simulink model "Model"  (R2020b)
settings: Solver=VariableStepAuto  StartTime=0.0  StopTime=20  MaxStep=0.1  RelTol=1e-1
values from neighbouring files (symbols this model uses):
  D = [0 ... (first row only)    [Data_clean.m]
  g = 9.81    [Data_clean.m]
  k_cart = 0.0113    [Data_clean.m]
  L = 5    [Data_clean.m]
  m = 12000    [Data_clean.m]
  M = 1000    [Data_clean.m]
  Ts = 0.1    [Data_clean.m]
undefined symbols (not defined in the file or in its folder): blk, Discrete, iA, isLTV, lastPcov, lastu, lastx, MDscale, mpc1_plant, MVscale, nCC, nu, nud, nv, nxp, ny, nym, p, RMVscale, Time, ts, uoff, X, xoff, Y, Yscale, Z
libraries: sm_lib x76, mpcsigdimcheck_private x76, nesl_utility x12, ctrlSharedLib x8, simulink_extras x5, mpclib x1
(part 1 of 8)
settings Model: Creator=kashirin.as  LastModifiedBy=LASK
settings SolverCC: AlgebraicLoopSolver=LineSearch
settings DebuggingCC: UnderSpecifiedDimensionMsg=warning
settings ConfigComp: PLC_TargetIDE=tiaportal_double

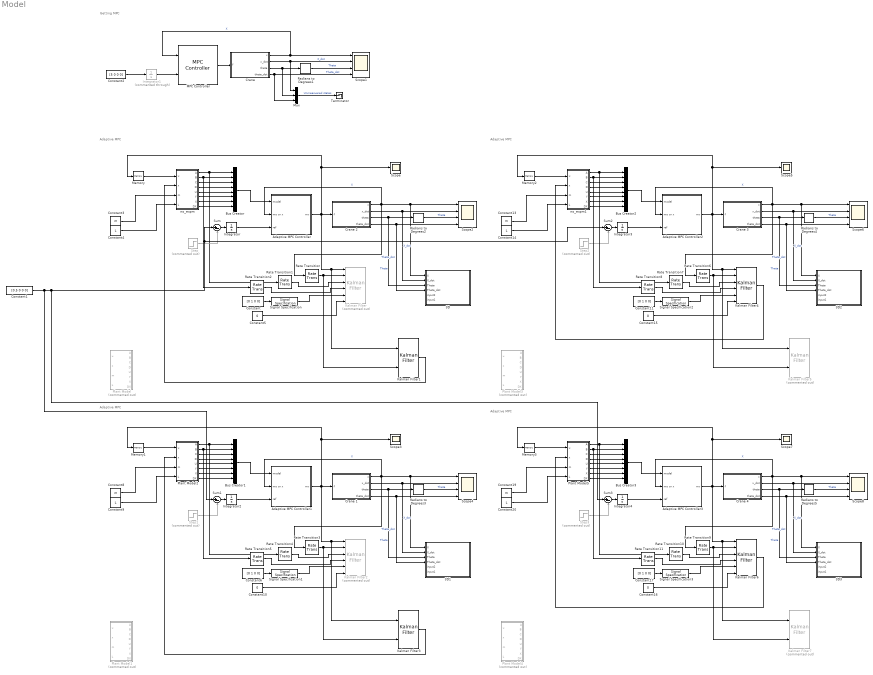
== system Model ==
  note: Getting MPC
  note: Adaptive MPC
  note: Adaptive MPC
  note: Adaptive MPC
  note: Adaptive MPC
  3D : Subsystem
  3D1 : Subsystem
  3D2 : Subsystem
  3D3 : Subsystem
  Adaptive MPC Controller : Subsystem  AncestorBlock=mpclib/Adaptive MPC Controller  SCDEnableBlockLinearizationSpecification=on  InitFcn=ampcblock_InitFcn  StartFcn=ampcblock_StartFcn  mask(Adaptive MPC){mpcobj=mpc1, x0=, enable_value=0, updateMPCinCallerWorkspace=on, md_inport=off, mv_inport=off, uref_inport=off, return_cost=off, return_mvseq=off, return_qpstatus=off, return_xseq=off, return_state=off, return_ovseq=off, state_inport=off, isltv_plant=off, umin_inport=off, umax_inport=off, ymin_inport=off, ymax_inport=off, cc_inport=off, ywt_inport=off, uwt_inport=off, duwt_inport=off, rhoeps_inport=off, pm_inport=off, MaximumP=10, HorizonChoice=FixedHorizon, BlockDataType=double, SampleTimeInherited=off, switch_inport=off}
      mask prompts: mpcobj "MPC:general:BlgAMPC"; x0 "MPC:general:BlgState"; enable_value "Value enabling optimization"; updateMPCinCallerWorkspace "Update MPC object in caller workspace"; md_inport "MPC:general:BlgMD"; mv_inport "MPC:general:BlgEXTMV"; uref_inport "MPC:general:BlgMVTARGET"; return_cost "MPC:general:BlgCOST"; return_mvseq "MPC:general:BlgMVSEQ"; return_qpstatus "MPC:general:BlgQPSTATUS"; return_xseq "MPC:general:BlgXSEQ"; return_state "MPC:general:BlgESTSTATE"; return_ovseq "MPC:general:BlgOVSEQ"; state_inport "MPC:general:BlgXKK"; isltv_plant "MPC:general:BlgLTV"; umin_inport "MPC:general:BlgMVMin"; umax_inport "MPC:general:BlgMVMax"; ymin_inport "MPC:general:BlgOVMin"; ymax_inport "MPC:general:BlgOVMax"; cc_inport "Custom constraints (E, F, G, S)"; ywt_inport "MPC:general:BlgYWT"; uwt_inport "MPC:general:BlgUWT"; duwt_inport "MPC:general:BlgDUWT"; rhoeps_inport "MPC:general:BlgECRWT"; pm_inport "MPC:general:BlgPM"; MaximumP "MPC:general:BlgMaximumP"; HorizonChoice "Simulink:Variants:LabelComboBox"; BlockDataType "MPC:general:BlgDATATYPE"; SampleTimeInherited "MPC:general:BlgTS"; switch_inport "MPC:general:BlgSWITCH"
      mask help: MPC:utility:MaskDescAdaptiveMPC1
      mask init:
      | [blk,ts,A,B,C,D,isQP,strmoorx,nmoorx,nu,nv,ny,nx,nym,nud,...
      |     degrees,lastPcov,H,Hinv,Linv,iA,Ac,Kx,Ku1,Kut,Kr,Kv,...
      |     Mlim,Mx,Mu1,Mv,z_degrees,utarget,...
      |     lastx,lastu,p,xoff,uoff,yoff,voff,myoff,no_md,no_ref,...
      |     CustomSolver,CustomSolverCodeGen,UseSuboptimalSolution,...
      |     UseActiveSetSolver,ASOptions,IPOptions,...
      |     nxQP,openloopflag,no_ym,no_mv,no_uref,...
      |     no_umin,no_umax,no_ymin,no_ymax,no_cc,...
      |     no_switch,CustomEstimation,...
      |     no_ywt, no_uwt, no_duwt, no_rhoeps,...
      |     Wy,Wdu,Jm,SuJm,Su1,Sx,Hv,Wu,I1,...
      |     isAdaptive, isLTV, Mrows, nCC, Ecc, Fcc, Scc, Gcc, Cid, Did, ...
      |     nxp, nup, nxid, mvindex, mdindex, unindex, myindex, ...
      |     Uscale, Yscale, MVscale, MDscale, ...
      |     RYscale,RMYscale,RMVscale,RMDscale,no_p,no_m,p0,m] = ampcblock_MaskInitFcnParameter();
      | ampcblock_MaskInitFcnResize(gcb,nv,nu,ny,nCC);
      mask Help: eval('mpcCSHelp(''MPCmaskAdaptive'',''HelpBrowser'')');
      mask Callback pm_inport: mpcblocks_callbackPM(gcb);
      mask TypeOptions HorizonChoice: MPC/optimizer/LabelModeActiveChoice
      mask DialogControl mpcobj Prompt: Adaptive MPC Controller
      mask DialogControl x0 Prompt: Initial Controller State
      mask DialogControl Container5 Prompt: MPC:general:BlgTab1
      mask DialogControl Container6 Prompt: MPC:general:BlgBox11
      mask DialogControl md_inport Prompt: Measured disturbance (md)
      mask DialogControl mv_inport Prompt: External manipulated variable (ext.mv)
      mask DialogControl uref_inport Prompt: Targets for manipulated variables (mv.target)
      mask DialogControl Container7 Prompt: MPC:general:BlgBox12
      mask DialogControl return_cost Prompt: Optimal cost (cost)
      mask DialogControl return_mvseq Prompt: Optimal control sequence (mv.seq)
      mask DialogControl return_qpstatus Prompt: Optimization status (qp.status)
      mask DialogControl return_xseq Prompt: Optimal state sequence (x.seq)
      mask DialogControl return_state Prompt: Estimated controller states (est.state)
      mask DialogControl return_ovseq Prompt: Optimal output sequence (y.seq)
      mask DialogControl Container16 Prompt: MPC:general:BlgBox13
      mask DialogControl state_inport Prompt: Use custom state estimation instead of using the built-in Kalman filter (x[k|k])
      mask DialogControl Container9 Prompt: MPC:general:BlgTab2
      mask DialogControl Container19 Prompt: MPC:general:BlgBox20
      mask DialogControl isltv_plant Prompt: Linear Time-Varying (LTV) plants (model expects 3-D signals)
      mask DialogControl Container10 Prompt: MPC:general:BlgBox21
      mask DialogControl umin_inport Prompt: Lower MV limits (umin)
      mask DialogControl umax_inport Prompt: Upper MV limits (umax)
      mask DialogControl ymin_inport Prompt: Lower OV limits (ymin)
      mask DialogControl ymax_inport Prompt: Upper OV limits (ymax)
      mask DialogControl Container11 Prompt: MPC:general:BlgBox22
      mask DialogControl ywt_inport Prompt: OV weights (y.wt)
      mask DialogControl uwt_inport Prompt: MV weights (u.wt)
      mask DialogControl duwt_inport Prompt: MVRate weights (du.wt)
      mask DialogControl rhoeps_inport Prompt: Slack variable weight (ecr.wt)
      mask DialogControl Container17 Prompt: Prediction and Control Horizons
      mask DialogControl pm_inport Prompt: Adjust prediction horizon (p) and control horizon (m) at run time
      mask DialogControl MaximumP Prompt: Maximum prediction horizon
      mask DialogControl HorizonChoice Prompt: Label mode active choice:
      mask DialogControl Container13 Prompt: MPC:general:BlgTab3
      mask DialogControl Container14 Prompt: MPC:general:BlgBox31
      mask DialogControl BlockDataType Prompt: Block Data Type
      mask DialogControl Container15 Prompt: MPC:general:BlgBox32
      mask DialogControl SampleTimeInherited Prompt: Inherit sample time (must be the same as controller sample time)
      mask DialogControl Container18 Prompt: MPC:general:BlgBox33
      mask DialogControl switch_inport Prompt: Use external signal to enable or disable optimization (switch)
      mask Display:
      | fprintf('Adaptive\nMPC');
      | port_label('output', 1, 'mv')
      | port_label('input', 1, 'model')
      | port_label('input', 2, 'mo')
      | port_label('input', 3, 'ref')
  Adaptive MPC Controller1 : Subsystem  AncestorBlock=mpclib/Adaptive MPC Controller  SCDEnableBlockLinearizationSpecification=on  InitFcn=ampcblock_InitFcn  StartFcn=ampcblock_StartFcn  mask(Adaptive MPC){mpcobj=mpc1, x0=, enable_value=0, updateMPCinCallerWorkspace=on, md_inport=off, mv_inport=off, uref_inport=off, return_cost=off, return_mvseq=off, return_qpstatus=off, return_xseq=off, return_state=off, return_ovseq=off, state_inport=off, isltv_plant=off, umin_inport=off, umax_inport=off, ymin_inport=off, ymax_inport=off, cc_inport=off, ywt_inport=off, uwt_inport=off, duwt_inport=off, rhoeps_inport=off, pm_inport=off, MaximumP=10, HorizonChoice=FixedHorizon, BlockDataType=double, SampleTimeInherited=off, switch_inport=off}
      mask prompts: mpcobj "MPC:general:BlgAMPC"; x0 "MPC:general:BlgState"; enable_value "Value enabling optimization"; updateMPCinCallerWorkspace "Update MPC object in caller workspace"; md_inport "MPC:general:BlgMD"; mv_inport "MPC:general:BlgEXTMV"; uref_inport "MPC:general:BlgMVTARGET"; return_cost "MPC:general:BlgCOST"; return_mvseq "MPC:general:BlgMVSEQ"; return_qpstatus "MPC:general:BlgQPSTATUS"; return_xseq "MPC:general:BlgXSEQ"; return_state "MPC:general:BlgESTSTATE"; return_ovseq "MPC:general:BlgOVSEQ"; state_inport "MPC:general:BlgXKK"; isltv_plant "MPC:general:BlgLTV"; umin_inport "MPC:general:BlgMVMin"; umax_inport "MPC:general:BlgMVMax"; ymin_inport "MPC:general:BlgOVMin"; ymax_inport "MPC:general:BlgOVMax"; cc_inport "Custom constraints (E, F, G, S)"; ywt_inport "MPC:general:BlgYWT"; uwt_inport "MPC:general:BlgUWT"; duwt_inport "MPC:general:BlgDUWT"; rhoeps_inport "MPC:general:BlgECRWT"; pm_inport "MPC:general:BlgPM"; MaximumP "MPC:general:BlgMaximumP"; HorizonChoice "Simulink:Variants:LabelComboBox"; BlockDataType "MPC:general:BlgDATATYPE"; SampleTimeInherited "MPC:general:BlgTS"; switch_inport "MPC:general:BlgSWITCH"
      mask help: MPC:utility:MaskDescAdaptiveMPC1
      mask init: same as Model/Adaptive MPC Controller
      mask Help: eval('mpcCSHelp(''MPCmaskAdaptive'',''HelpBrowser'')');
      mask Callback pm_inport: mpcblocks_callbackPM(gcb);
      mask TypeOptions HorizonChoice: MPC/optimizer/LabelModeActiveChoice
      mask DialogControl mpcobj Prompt: Adaptive MPC Controller
      mask DialogControl x0 Prompt: Initial Controller State
      mask DialogControl Container5 Prompt: MPC:general:BlgTab1
      mask DialogControl Container6 Prompt: MPC:general:BlgBox11
      mask DialogControl md_inport Prompt: Measured disturbance (md)
      mask DialogControl mv_inport Prompt: External manipulated variable (ext.mv)
      mask DialogControl uref_inport Prompt: Targets for manipulated variables (mv.target)
      mask DialogControl Container7 Prompt: MPC:general:BlgBox12
      mask DialogControl return_cost Prompt: Optimal cost (cost)
      mask DialogControl return_mvseq Prompt: Optimal control sequence (mv.seq)
      mask DialogControl return_qpstatus Prompt: Optimization status (qp.status)
      mask DialogControl return_xseq Prompt: Optimal state sequence (x.seq)
      mask DialogControl return_state Prompt: Estimated controller states (est.state)
      mask DialogControl return_ovseq Prompt: Optimal output sequence (y.seq)
      mask DialogControl Container16 Prompt: MPC:general:BlgBox13
      mask DialogControl state_inport Prompt: Use custom state estimation instead of using the built-in Kalman filter (x[k|k])
      mask DialogControl Container9 Prompt: MPC:general:BlgTab2
      mask DialogControl Container19 Prompt: MPC:general:BlgBox20
      mask DialogControl isltv_plant Prompt: Linear Time-Varying (LTV) plants (model expects 3-D signals)
      mask DialogControl Container10 Prompt: MPC:general:BlgBox21
      mask DialogControl umin_inport Prompt: Lower MV limits (umin)
      mask DialogControl umax_inport Prompt: Upper MV limits (umax)
      mask DialogControl ymin_inport Prompt: Lower OV limits (ymin)
      mask DialogControl ymax_inport Prompt: Upper OV limits (ymax)
      mask DialogControl Container11 Prompt: MPC:general:BlgBox22
      mask DialogControl ywt_inport Prompt: OV weights (y.wt)
      mask DialogControl uwt_inport Prompt: MV weights (u.wt)
      mask DialogControl duwt_inport Prompt: MVRate weights (du.wt)
      mask DialogControl rhoeps_inport Prompt: Slack variable weight (ecr.wt)
      mask DialogControl Container17 Prompt: Prediction and Control Horizons
      mask DialogControl pm_inport Prompt: Adjust prediction horizon (p) and control horizon (m) at run time
      mask DialogControl MaximumP Prompt: Maximum prediction horizon
      mask DialogControl HorizonChoice Prompt: Label mode active choice:
      mask DialogControl Container13 Prompt: MPC:general:BlgTab3
      mask DialogControl Container14 Prompt: MPC:general:BlgBox31
      mask DialogControl BlockDataType Prompt: Block Data Type
      mask DialogControl Container15 Prompt: MPC:general:BlgBox32
      mask DialogControl SampleTimeInherited Prompt: Inherit sample time (must be the same as controller sample time)
      mask DialogControl Container18 Prompt: MPC:general:BlgBox33
      mask DialogControl switch_inport Prompt: Use external signal to enable or disable optimization (switch)
      mask Display:
      | fprintf('Adaptive\nMPC');
      | port_label('output', 1, 'mv')
      | port_label('input', 1, 'model')
      | port_label('input', 2, 'mo')
      | port_label('input', 3, 'ref')
  Adaptive MPC Controller2 : Subsystem  AncestorBlock=mpclib/Adaptive MPC Controller  SCDEnableBlockLinearizationSpecification=on  InitFcn=ampcblock_InitFcn  StartFcn=ampcblock_StartFcn  mask(Adaptive MPC){mpcobj=mpc1, x0=, enable_value=0, updateMPCinCallerWorkspace=on, md_inport=off, mv_inport=off, uref_inport=off, return_cost=off, return_mvseq=off, return_qpstatus=off, return_xseq=off, return_state=off, return_ovseq=off, state_inport=off, isltv_plant=off, umin_inport=off, umax_inport=off, ymin_inport=off, ymax_inport=off, cc_inport=off, ywt_inport=off, uwt_inport=off, duwt_inport=off, rhoeps_inport=off, pm_inport=off, MaximumP=10, HorizonChoice=FixedHorizon, BlockDataType=double, SampleTimeInherited=off, switch_inport=off}
      mask prompts: mpcobj "MPC:general:BlgAMPC"; x0 "MPC:general:BlgState"; enable_value "Value enabling optimization"; updateMPCinCallerWorkspace "Update MPC object in caller workspace"; md_inport "MPC:general:BlgMD"; mv_inport "MPC:general:BlgEXTMV"; uref_inport "MPC:general:BlgMVTARGET"; return_cost "MPC:general:BlgCOST"; return_mvseq "MPC:general:BlgMVSEQ"; return_qpstatus "MPC:general:BlgQPSTATUS"; return_xseq "MPC:general:BlgXSEQ"; return_state "MPC:general:BlgESTSTATE"; return_ovseq "MPC:general:BlgOVSEQ"; state_inport "MPC:general:BlgXKK"; isltv_plant "MPC:general:BlgLTV"; umin_inport "MPC:general:BlgMVMin"; umax_inport "MPC:general:BlgMVMax"; ymin_inport "MPC:general:BlgOVMin"; ymax_inport "MPC:general:BlgOVMax"; cc_inport "Custom constraints (E, F, G, S)"; ywt_inport "MPC:general:BlgYWT"; uwt_inport "MPC:general:BlgUWT"; duwt_inport "MPC:general:BlgDUWT"; rhoeps_inport "MPC:general:BlgECRWT"; pm_inport "MPC:general:BlgPM"; MaximumP "MPC:general:BlgMaximumP"; HorizonChoice "Simulink:Variants:LabelComboBox"; BlockDataType "MPC:general:BlgDATATYPE"; SampleTimeInherited "MPC:general:BlgTS"; switch_inport "MPC:general:BlgSWITCH"
      mask help: MPC:utility:MaskDescAdaptiveMPC1
      mask init: same as Model/Adaptive MPC Controller
      mask Help: eval('mpcCSHelp(''MPCmaskAdaptive'',''HelpBrowser'')');
      mask Callback pm_inport: mpcblocks_callbackPM(gcb);
      mask TypeOptions HorizonChoice: MPC/optimizer/LabelModeActiveChoice
      mask DialogControl mpcobj Prompt: Adaptive MPC Controller
      mask DialogControl x0 Prompt: Initial Controller State
      mask DialogControl Container5 Prompt: MPC:general:BlgTab1
      mask DialogControl Container6 Prompt: MPC:general:BlgBox11
      mask DialogControl md_inport Prompt: Measured disturbance (md)
      mask DialogControl mv_inport Prompt: External manipulated variable (ext.mv)
      mask DialogControl uref_inport Prompt: Targets for manipulated variables (mv.target)
      mask DialogControl Container7 Prompt: MPC:general:BlgBox12
      mask DialogControl return_cost Prompt: Optimal cost (cost)
      mask DialogControl return_mvseq Prompt: Optimal control sequence (mv.seq)
      mask DialogControl return_qpstatus Prompt: Optimization status (qp.status)
      mask DialogControl return_xseq Prompt: Optimal state sequence (x.seq)
      mask DialogControl return_state Prompt: Estimated controller states (est.state)
      mask DialogControl return_ovseq Prompt: Optimal output sequence (y.seq)
      mask DialogControl Container16 Prompt: MPC:general:BlgBox13
      mask DialogControl state_inport Prompt: Use custom state estimation instead of using the built-in Kalman filter (x[k|k])
      mask DialogControl Container9 Prompt: MPC:general:BlgTab2
      mask DialogControl Container19 Prompt: MPC:general:BlgBox20
      mask DialogControl isltv_plant Prompt: Linear Time-Varying (LTV) plants (model expects 3-D signals)
      mask DialogControl Container10 Prompt: MPC:general:BlgBox21
      mask DialogControl umin_inport Prompt: Lower MV limits (umin)
      mask DialogControl umax_inport Prompt: Upper MV limits (umax)
      mask DialogControl ymin_inport Prompt: Lower OV limits (ymin)
      mask DialogControl ymax_inport Prompt: Upper OV limits (ymax)
      mask DialogControl Container11 Prompt: MPC:general:BlgBox22
      mask DialogControl ywt_inport Prompt: OV weights (y.wt)
      mask DialogControl uwt_inport Prompt: MV weights (u.wt)
      mask DialogControl duwt_inport Prompt: MVRate weights (du.wt)
      mask DialogControl rhoeps_inport Prompt: Slack variable weight (ecr.wt)
      mask DialogControl Container17 Prompt: Prediction and Control Horizons
      mask DialogControl pm_inport Prompt: Adjust prediction horizon (p) and control horizon (m) at run time
      mask DialogControl MaximumP Prompt: Maximum prediction horizon
      mask DialogControl HorizonChoice Prompt: Label mode active choice:
      mask DialogControl Container13 Prompt: MPC:general:BlgTab3
      mask DialogControl Container14 Prompt: MPC:general:BlgBox31
      mask DialogControl BlockDataType Prompt: Block Data Type
      mask DialogControl Container15 Prompt: MPC:general:BlgBox32
      mask DialogControl SampleTimeInherited Prompt: Inherit sample time (must be the same as controller sample time)
      mask DialogControl Container18 Prompt: MPC:general:BlgBox33
      mask DialogControl switch_inport Prompt: Use external signal to enable or disable optimization (switch)
      mask Display:
      | fprintf('Adaptive\nMPC');
      | port_label('output', 1, 'mv')
      | port_label('input', 1, 'model')
      | port_label('input', 2, 'mo')
      | port_label('input', 3, 'ref')
  Adaptive MPC Controller3 : Subsystem  AncestorBlock=mpclib/Adaptive MPC Controller  SCDEnableBlockLinearizationSpecification=on  InitFcn=ampcblock_InitFcn  StartFcn=ampcblock_StartFcn  mask(Adaptive MPC){mpcobj=mpc1, x0=, enable_value=0, updateMPCinCallerWorkspace=on, md_inport=off, mv_inport=off, uref_inport=off, return_cost=off, return_mvseq=off, return_qpstatus=off, return_xseq=off, return_state=off, return_ovseq=off, state_inport=off, isltv_plant=off, umin_inport=off, umax_inport=off, ymin_inport=off, ymax_inport=off, cc_inport=off, ywt_inport=off, uwt_inport=off, duwt_inport=off, rhoeps_inport=off, pm_inport=off, MaximumP=10, HorizonChoice=FixedHorizon, BlockDataType=double, SampleTimeInherited=off, switch_inport=off}
      mask prompts: mpcobj "MPC:general:BlgAMPC"; x0 "MPC:general:BlgState"; enable_value "Value enabling optimization"; updateMPCinCallerWorkspace "Update MPC object in caller workspace"; md_inport "MPC:general:BlgMD"; mv_inport "MPC:general:BlgEXTMV"; uref_inport "MPC:general:BlgMVTARGET"; return_cost "MPC:general:BlgCOST"; return_mvseq "MPC:general:BlgMVSEQ"; return_qpstatus "MPC:general:BlgQPSTATUS"; return_xseq "MPC:general:BlgXSEQ"; return_state "MPC:general:BlgESTSTATE"; return_ovseq "MPC:general:BlgOVSEQ"; state_inport "MPC:general:BlgXKK"; isltv_plant "MPC:general:BlgLTV"; umin_inport "MPC:general:BlgMVMin"; umax_inport "MPC:general:BlgMVMax"; ymin_inport "MPC:general:BlgOVMin"; ymax_inport "MPC:general:BlgOVMax"; cc_inport "Custom constraints (E, F, G, S)"; ywt_inport "MPC:general:BlgYWT"; uwt_inport "MPC:general:BlgUWT"; duwt_inport "MPC:general:BlgDUWT"; rhoeps_inport "MPC:general:BlgECRWT"; pm_inport "MPC:general:BlgPM"; MaximumP "MPC:general:BlgMaximumP"; HorizonChoice "Simulink:Variants:LabelComboBox"; BlockDataType "MPC:general:BlgDATATYPE"; SampleTimeInherited "MPC:general:BlgTS"; switch_inport "MPC:general:BlgSWITCH"
      mask help: MPC:utility:MaskDescAdaptiveMPC1
      mask init: same as Model/Adaptive MPC Controller
      mask Help: eval('mpcCSHelp(''MPCmaskAdaptive'',''HelpBrowser'')');
      mask Callback pm_inport: mpcblocks_callbackPM(gcb);
      mask TypeOptions HorizonChoice: MPC/optimizer/LabelModeActiveChoice
      mask DialogControl mpcobj Prompt: Adaptive MPC Controller
      mask DialogControl x0 Prompt: Initial Controller State
      mask DialogControl Container5 Prompt: MPC:general:BlgTab1
      mask DialogControl Container6 Prompt: MPC:general:BlgBox11
      mask DialogControl md_inport Prompt: Measured disturbance (md)
      mask DialogControl mv_inport Prompt: External manipulated variable (ext.mv)
      mask DialogControl uref_inport Prompt: Targets for manipulated variables (mv.target)
      mask DialogControl Container7 Prompt: MPC:general:BlgBox12
      mask DialogControl return_cost Prompt: Optimal cost (cost)
      mask DialogControl return_mvseq Prompt: Optimal control sequence (mv.seq)
      mask DialogControl return_qpstatus Prompt: Optimization status (qp.status)
      mask DialogControl return_xseq Prompt: Optimal state sequence (x.seq)
      mask DialogControl return_state Prompt: Estimated controller states (est.state)
      mask DialogControl return_ovseq Prompt: Optimal output sequence (y.seq)
      mask DialogControl Container16 Prompt: MPC:general:BlgBox13
      mask DialogControl state_inport Prompt: Use custom state estimation instead of using the built-in Kalman filter (x[k|k])
      mask DialogControl Container9 Prompt: MPC:general:BlgTab2
      mask DialogControl Container19 Prompt: MPC:general:BlgBox20
      mask DialogControl isltv_plant Prompt: Linear Time-Varying (LTV) plants (model expects 3-D signals)
      mask DialogControl Container10 Prompt: MPC:general:BlgBox21
      mask DialogControl umin_inport Prompt: Lower MV limits (umin)
      mask DialogControl umax_inport Prompt: Upper MV limits (umax)
      mask DialogControl ymin_inport Prompt: Lower OV limits (ymin)
      mask DialogControl ymax_inport Prompt: Upper OV limits (ymax)
      mask DialogControl Container11 Prompt: MPC:general:BlgBox22
      mask DialogControl ywt_inport Prompt: OV weights (y.wt)
      mask DialogControl uwt_inport Prompt: MV weights (u.wt)
      mask DialogControl duwt_inport Prompt: MVRate weights (du.wt)
      mask DialogControl rhoeps_inport Prompt: Slack variable weight (ecr.wt)
      mask DialogControl Container17 Prompt: Prediction and Control Horizons
      mask DialogControl pm_inport Prompt: Adjust prediction horizon (p) and control horizon (m) at run time
      mask DialogControl MaximumP Prompt: Maximum prediction horizon
      mask DialogControl HorizonChoice Prompt: Label mode active choice:
      mask DialogControl Container13 Prompt: MPC:general:BlgTab3
      mask DialogControl Container14 Prompt: MPC:general:BlgBox31
      mask DialogControl BlockDataType Prompt: Block Data Type
      mask DialogControl Container15 Prompt: MPC:general:BlgBox32
      mask DialogControl SampleTimeInherited Prompt: Inherit sample time (must be the same as controller sample time)
      mask DialogControl Container18 Prompt: MPC:general:BlgBox33
      mask DialogControl switch_inport Prompt: Use external signal to enable or disable optimization (switch)
      mask Display:
      | fprintf('Adaptive\nMPC');
      | port_label('output', 1, 'mv')
      | port_label('input', 1, 'model')
      | port_label('input', 2, 'mo')
      | port_label('input', 3, 'ref')
  Bus Creator{,1..3} (4 alike) : BusCreator  Inputs=8
  Constant{,6,11,17} (4 alike) : Constant  Value=[0 1 0 0]
  Constant1 : Constant  Value=[0.5 0 0 0]
  Constant{5,10,15..16} (4 alike) : Constant  Value=0
  Constant{3,8,13,19} (4 alike) : Constant  Value=m
  Constant{4,9,14,20} (4 alike) : Constant  Value=L
  Constant2 : Constant  Value=[5 0 0 0]
  Crane : Subsystem
  Crane 1 : Subsystem
  Crane 2 : Subsystem
  Crane 3 : Subsystem
  Crane 4 : Subsystem
  Integrator{,2..4} (4 alike) : Integrator
  Integrator1 : Integrator  Commented=through
  Kalman Filter : ctrlSharedLib/Kalman Filter  Commented=on  TimeDomain=Discrete-Time  UseCurrentEstimator=on  ModelSource=Input port  ModelSourceVariable=ss(0.95,1,1,0,1)  A=mpc1_plant.A  B=mpc1_plant.B  C=[0 1 0 0]  D=0  NumberOfStates=4  NumberOfInputs=1  NumberOfOutputs=1  InitialEstimateSource=Dialog  X0=[0 0 0 0]  P0=10  UseK=off  UseGH=off  NumberOfProcessNoiseInputs=1  G=1  TimeInvariantG=on  H=0  TimeInvariantH=on  Q=0.05  TimeInvariantQ=on  R=1  TimeInvariantR=on  N=0  TimeInvariantN=on  AddInputPort=on  AddEnablePort=off  OutputEstimatedY=off  OutputP=off  Ts=Ts
  Kalman Filter1 : ctrlSharedLib/Kalman Filter  TimeDomain=Discrete-Time  UseCurrentEstimator=on  ModelSource=Individual A, B, C, D matrices  ModelSourceVariable=ss(0.95,1,1,0,1)  A=mpc1_plant.A  B=mpc1_plant.B  C=[0 1 0 0]  D=0  NumberOfStates=4  NumberOfInputs=1  NumberOfOutputs=1  InitialEstimateSource=Dialog  X0=[0 0 0 0]  P0=10  UseK=off  UseGH=off  NumberOfProcessNoiseInputs=1  G=1  TimeInvariantG=on  H=0  TimeInvariantH=on  Q=0.05  TimeInvariantQ=on  R=1  TimeInvariantR=on  N=0  TimeInvariantN=on  AddInputPort=on  AddEnablePort=off  OutputEstimatedY=off  OutputP=off  Ts=Ts
  Kalman Filter2 : ctrlSharedLib/Kalman Filter  Commented=on  TimeDomain=Discrete-Time  UseCurrentEstimator=on  ModelSource=Input port  ModelSourceVariable=ss(0.95,1,1,0,1)  A=mpc1_plant.A  B=mpc1_plant.B  C=[0 1 0 0]  D=0  NumberOfStates=4  NumberOfInputs=1  NumberOfOutputs=1  InitialEstimateSource=Dialog  X0=[0 0 0 0]  P0=10  UseK=off  UseGH=off  NumberOfProcessNoiseInputs=1  G=1  TimeInvariantG=on  H=0  TimeInvariantH=on  Q=0.05  TimeInvariantQ=on  R=1  TimeInvariantR=on  N=0  TimeInvariantN=on  AddInputPort=on  AddEnablePort=off  OutputEstimatedY=off  OutputP=off  Ts=Ts
  Kalman Filter3 : ctrlSharedLib/Kalman Filter  TimeDomain=Discrete-Time  UseCurrentEstimator=on  ModelSource=Individual A, B, C, D matrices  ModelSourceVariable=ss(0.95,1,1,0,1)  A=mpc1_plant.A  B=mpc1_plant.B  C=[0 1 0 0]  D=0  NumberOfStates=4  NumberOfInputs=1  NumberOfOutputs=1  InitialEstimateSource=Dialog  X0=[0 0 0 0]  P0=10  UseK=off  UseGH=off  NumberOfProcessNoiseInputs=1  G=1  TimeInvariantG=on  H=0  TimeInvariantH=on  Q=0.05  TimeInvariantQ=on  R=1  TimeInvariantR=on  N=0  TimeInvariantN=on  AddInputPort=on  AddEnablePort=off  OutputEstimatedY=off  OutputP=off  Ts=Ts
  Kalman Filter4 : ctrlSharedLib/Kalman Filter  TimeDomain=Discrete-Time  UseCurrentEstimator=on  ModelSource=Input port  ModelSourceVariable=ss(0.95,1,1,0,1)  A=mpc1_plant.A  B=mpc1_plant.B  C=[0 1 0 0]  D=0  NumberOfStates=4  NumberOfInputs=1  NumberOfOutputs=1  InitialEstimateSource=Dialog  X0=[0 0 0 0]  P0=10  UseK=off  UseGH=off  NumberOfProcessNoiseInputs=1  G=1  TimeInvariantG=on  H=0  TimeInvariantH=on  Q=0.05  TimeInvariantQ=on  R=1  TimeInvariantR=on  N=0  TimeInvariantN=on  AddInputPort=on  AddEnablePort=off  OutputEstimatedY=off  OutputP=off  Ts=Ts
  Kalman Filter5 : ctrlSharedLib/Kalman Filter  Commented=on  TimeDomain=Discrete-Time  UseCurrentEstimator=on  ModelSource=Individual A, B, C, D matrices  ModelSourceVariable=ss(0.95,1,1,0,1)  A=mpc1_plant.A  B=mpc1_plant.B  C=[0 1 0 0]  D=0  NumberOfStates=4  NumberOfInputs=1  NumberOfOutputs=1  InitialEstimateSource=Dialog  X0=[0 0 0 0]  P0=10  UseK=off  UseGH=off  NumberOfProcessNoiseInputs=1  G=1  TimeInvariantG=on  H=0  TimeInvariantH=on  Q=0.05  TimeInvariantQ=on  R=1  TimeInvariantR=on  N=0  TimeInvariantN=on  AddInputPort=on  AddEnablePort=off  OutputEstimatedY=off  OutputP=off  Ts=Ts
  Kalman Filter6 : ctrlSharedLib/Kalman Filter  TimeDomain=Discrete-Time  UseCurrentEstimator=on  ModelSource=Input port  ModelSourceVariable=ss(0.95,1,1,0,1)  A=mpc1_plant.A  B=mpc1_plant.B  C=[0 1 0 0]  D=0  NumberOfStates=4  NumberOfInputs=1  NumberOfOutputs=1  InitialEstimateSource=Dialog  X0=[0 0 0 0]  P0=10  UseK=off  UseGH=off  NumberOfProcessNoiseInputs=1  G=1  TimeInvariantG=on  H=0  TimeInvariantH=on  Q=0.05  TimeInvariantQ=on  R=1  TimeInvariantR=on  N=0  TimeInvariantN=on  AddInputPort=on  AddEnablePort=off  OutputEstimatedY=off  OutputP=off  Ts=Ts
  Kalman Filter7 : ctrlSharedLib/Kalman Filter  Commented=on  TimeDomain=Discrete-Time  UseCurrentEstimator=on  ModelSource=Individual A, B, C, D matrices  ModelSourceVariable=ss(0.95,1,1,0,1)  A=mpc1_plant.A  B=mpc1_plant.B  C=[0 1 0 0]  D=0  NumberOfStates=4  NumberOfInputs=1  NumberOfOutputs=1  InitialEstimateSource=Dialog  X0=[0 0 0 0]  P0=10  UseK=off  UseGH=off  NumberOfProcessNoiseInputs=1  G=1  TimeInvariantG=on  H=0  TimeInvariantH=on  Q=0.05  TimeInvariantQ=on  R=1  TimeInvariantR=on  N=0  TimeInvariantN=on  AddInputPort=on  AddEnablePort=off  OutputEstimatedY=off  OutputP=off  Ts=Ts
  MPC Controller : mpclib/MPC Controller  SCDEnableBlockLinearizationSpecification=on  mpcobj=mpc1  is_multiple=0  enable_value=0  return_u0=off  updateMPCinCallerWorkspace=on  md_inport=off  mv_inport=off  uref_inport=off  return_cost=off  return_mvseq=off  return_qpstatus=off  return_xseq=off  return_state=off  return_ovseq=off  state_inport=off  umin_inport=off  umax_inport=off  ymin_inport=off  ymax_inport=off  cc_inport=off  ywt_inport=off  uwt_inport=off  duwt_inport=off  rhoeps_inport=off  pm_inport=off  MaximumP=10  HorizonChoice=FixedHorizon  n_ts=0.1  n_p=70  n_mv=1  n_md=0  n_ud=0  n_mo=1  n_uo=3  BlockDataType=double  SampleTimeInherited=off  switch_inport=off
  Memory{,1..3} (4 alike) : Memory
  Mux : Mux  Inputs=3
  Plant Model : MATLAB Function  Commented=on  TreatAsAtomicUnit=on
  Plant Model1 : MATLAB Function  Commented=on  TreatAsAtomicUnit=on
  Plant Model2 : MATLAB Function  TreatAsAtomicUnit=on
  Plant Model3 : MATLAB Function  Commented=on  TreatAsAtomicUnit=on
  Plant Model4 : MATLAB Function  Commented=on  TreatAsAtomicUnit=on
  Plant Model5 : MATLAB Function  TreatAsAtomicUnit=on
  Radians to Degrees{1..5} (5 alike) : simulink_extras/Transformations/Radians to Degrees
  Rate Transition{,1..11} (12 alike) : RateTransition  OutPortSampleTime=Ts
  Scope{,3,5,7} (4 alike) : Scope
  Scope{1..2,4,6,8} (5 alike) : Scope  NumInputPorts=4
  Signal Specification{,1..3} (4 alike) : SignalSpecification  Dimensions=[1 4]
  Step{,1..3} (4 alike) : Step  Commented=on  Time=5  After=[2 0 0 0]  SampleTime=0
  Sum{,1..3} (4 alike) : Sum  Inputs=|+-
  Terminator : Terminator
  no_expm : MATLAB Function  TreatAsAtomicUnit=on
  no_expm1 : MATLAB Function  TreatAsAtomicUnit=on
  wires:
  Adaptive MPC Controller/1(mv) -> Crane 2/1(f), Kalman Filter/1, Kalman Filter1/1, Scope/1, Memory/1
  no_expm/1(A) -> Bus Creator/1, Rate Transition1/1
  no_expm/3(C) -> Bus Creator/3
  no_expm/4(D) -> Bus Creator/4
  no_expm/8(DX) -> Bus Creator/8
  no_expm/6(Y) -> Bus Creator/6
  no_expm/5(U) -> Bus Creator/5
  no_expm/7(X) -> Bus Creator/7
  Memory/1 -> no_expm/1(u)
  Bus Creator/1 -> Adaptive MPC Controller/1(model)
  Crane 2/4(theta_dot) -> Scope2/4, 3D/4(Theta_dot)  "Theta_dot"
  Crane 2/1(x) -> Adaptive MPC Controller/2(mo or x), Scope2/1, 3D/1(X), Rate Transition/1  "X"
  Crane 2/3(theta) -> Radians to Degrees2/1, 3D/3(Theta)  "Theta"
  Crane 2/2(x_dot) -> Scope2/2, 3D/2(X_dot)  "X_dot"
  Constant3/1 -> no_expm/3(m)
  Constant4/1 -> no_expm/4(L)
  Rate Transition/1 -> Kalman Filter1/2, Kalman Filter/2
  Mux/1 -> Terminator/1  "Unmeasuared states"
  Radians to Degrees1/1 -> Scope1/3  "Theta"
  Crane/1(x) -> Scope1/1, MPC Controller/1  "X"
  Crane/2(x_dot) -> Scope1/2, Mux/1  "X_dot"
  Constant2/1 -> Integrator1/1
  MPC Controller/1 -> Crane/1(f)
  Integrator1/1 -> MPC Controller/2
  Crane/4(theta_dot) -> Mux/3, Scope1/4  "Theta_dot"
  Crane/3(theta) -> Radians to Degrees1/1, Mux/2
  Radians to Degrees2/1 -> Scope2/3  "Theta"
  Integrator/1 -> Adaptive MPC Controller/3(ref)
  Sum/1 -> Integrator/1
  Step/1 -> Sum/2
  Rate Transition1/1 -> Kalman Filter/3
  Rate Transition2/1 -> Kalman Filter/4
  Constant/1 -> Signal Specification/1
  Constant5/1 -> Kalman Filter/6
  Signal Specification/1 -> Kalman Filter/5
  Kalman Filter1/1 -> no_expm/2(x)
  Constant6/1 -> Signal Specification1/1
  Rate Transition5/1 -> Kalman Filter2/4
  Kalman Filter3/1 -> Plant Model2/2(x)
  Step1/1 -> Sum1/2
  Plant Model2/1(A) -> Bus Creator1/1, Rate Transition4/1
  Signal Specification1/1 -> Kalman Filter2/5
  Radians to Degrees3/1 -> Scope4/3  "Theta"
  Constant9/1 -> Plant Model2/4(L)
  Integrator2/1 -> Adaptive MPC Controller1/3(ref)
  Crane 1/4(theta_dot) -> Scope4/4, 3D1/4(Theta_dot)  "Theta_dot"
  Constant8/1 -> Plant Model2/3(m)
  Rate Transition3/1 -> Kalman Filter3/2, Kalman Filter2/2
  Crane 1/1(x) -> Adaptive MPC Controller1/2(mo or x), Scope4/1, 3D1/1(X), Rate Transition3/1  "X"
  Bus Creator1/1 -> Adaptive MPC Controller1/1(model)
  Memory1/1 -> Plant Model2/1(u)
  Rate Transition4/1 -> Kalman Filter2/3
  Crane 1/2(x_dot) -> Scope4/2, 3D1/2(X_dot)  "X_dot"
  Plant Model2/7(X) -> Bus Creator1/7
  Plant Model2/3(C) -> Bus Creator1/3
  Plant Model2/4(D) -> Bus Creator1/4
  Plant Model2/5(U) -> Bus Creator1/5
  Plant Model2/2(B) -> Bus Creator1/2, Rate Transition5/1
  Plant Model2/6(Y) -> Bus Creator1/6
  Adaptive MPC Controller1/1(mv) -> Crane 1/1(f), Kalman Filter2/1, Kalman Filter3/1, Scope3/1, Memory1/1
  Sum1/1 -> Integrator2/1
  Plant Model2/8(DX) -> Bus Creator1/8
  Constant10/1 -> Kalman Filter2/6
  Crane 1/3(theta) -> Radians to Degrees3/1, 3D1/3(Theta)  "Theta"
  Constant11/1 -> Signal Specification2/1
  Rate Transition8/1 -> Kalman Filter4/4
  Step2/1 -> Sum2/2
  no_expm1/1(A) -> Bus Creator2/1, Rate Transition7/1
  Signal Specification2/1 -> Kalman Filter4/5
  Radians to Degrees4/1 -> Scope6/3  "Theta"
  Constant14/1 -> no_expm1/4(L)
  Integrator3/1 -> Adaptive MPC Controller2/3(ref)
  Crane 3/4(theta_dot) -> Scope6/4, 3D2/4(Theta_dot)  "Theta_dot"
  Constant13/1 -> no_expm1/3(m)
  Rate Transition6/1 -> Kalman Filter5/2, Kalman Filter4/2
  Crane 3/1(x) -> Adaptive MPC Controller2/2(mo or x), Scope6/1, 3D2/1(X), Rate Transition6/1  "X"
  Bus Creator2/1 -> Adaptive MPC Controller2/1(model)
  Memory2/1 -> no_expm1/1(u)
  Rate Transition7/1 -> Kalman Filter4/3
  Crane 3/2(x_dot) -> Scope6/2, 3D2/2(X_dot)  "X_dot"
  no_expm1/7(X) -> Bus Creator2/7
  no_expm1/3(C) -> Bus Creator2/3
  no_expm1/4(D) -> Bus Creator2/4
  no_expm1/5(U) -> Bus Creator2/5
  no_expm1/2(B) -> Bus Creator2/2, Rate Transition8/1
  no_expm1/6(Y) -> Bus Creator2/6
  Adaptive MPC Controller2/1(mv) -> Crane 3/1(f), Kalman Filter4/1, Kalman Filter5/1, Scope5/1, Memory2/1
  Sum2/1 -> Integrator3/1
  no_expm1/8(DX) -> Bus Creator2/8
  no_expm/2(B) -> Bus Creator/2, Rate Transition2/1
  Constant15/1 -> Kalman Filter4/6
  Crane 3/3(theta) -> Radians to Degrees4/1, 3D2/3(Theta)  "Theta"
  Kalman Filter4/1 -> no_expm1/2(x)
  Crane 4/1(x) -> Adaptive MPC Controller3/2(mo or x), Scope8/1, 3D3/1(X), Rate Transition9/1  "X"
  Adaptive MPC Controller3/1(mv) -> Crane 4/1(f), Kalman Filter6/1, Kalman Filter7/1, Scope7/1, Memory3/1
  Crane 4/3(theta) -> Radians to Degrees5/1, 3D3/3(Theta)  "Theta"
  Crane 4/2(x_dot) -> Scope8/2, 3D3/2(X_dot)  "X_dot"
  Rate Transition10/1 -> Kalman Filter6/3
  Constant16/1 -> Kalman Filter6/6
  Rate Transition9/1 -> Kalman Filter7/2, Kalman Filter6/2
  Integrator4/1 -> Adaptive MPC Controller3/3(ref)
  Bus Creator3/1 -> Adaptive MPC Controller3/1(model)
  Sum3/1 -> Integrator4/1
  Radians to Degrees5/1 -> Scope8/3  "Theta"
  Step3/1 -> Sum3/2
  Signal Specification3/1 -> Kalman Filter6/5
  Rate Transition11/1 -> Kalman Filter6/4
  Constant17/1 -> Signal Specification3/1
  Memory3/1 -> Plant Model5/1(u)
  Plant Model5/1(A) -> Bus Creator3/1, Rate Transition10/1
  Constant20/1 -> Plant Model5/4(L)
  Plant Model5/2(B) -> Bus Creator3/2, Rate Transition11/1
  Crane 4/4(theta_dot) -> Scope8/4, 3D3/4(Theta_dot)  "Theta_dot"
  Plant Model5/5(U) -> Bus Creator3/5
  Constant1/1 -> Sum1/1, Sum3/1, Sum/1, Sum2/1
  Plant Model5/3(C) -> Bus Creator3/3
  Constant19/1 -> Plant Model5/3(m)
  Plant Model5/4(D) -> Bus Creator3/4
  Plant Model5/7(X) -> Bus Creator3/7
  Plant Model5/8(DX) -> Bus Creator3/8
  Plant Model5/6(Y) -> Bus Creator3/6
  Kalman Filter6/1 -> Plant Model5/2(x)
